simulink model "GraphicalFunction3_2018a"  (R2018a)
settings: Solver=FixedStepDiscrete  StartTime=0.0  StopTime=0.1  FixedStep=0.1  RelTol=1e-3  EnableMultiTasking=on
settings Model: Creator=bzhan  LastModifiedBy=bzhan
settings SolverCC: AutoInsertRateTranBlk=on
settings DataIOCC: LimitDataPoints=on  ReturnWorkspaceOutputs=on
settings OptimizationCC: LifeSpan=inf
settings DebuggingCC: AllowSymbolicDim=off  SFUnexpectedBacktrackingDiag=warning  SFNoUnconditionalDefaultTransitionDiag=warning  SFExecutionAtInitializationDiag=none
settings CodeAppCC: StateflowObjectComments=on
settings GRTTargetCC: TargetLangStandard=C89/C90 (ANSI)
settings ConfigComp: CovMetricSettings=dw  CovHtmlReporting=on  CovSaveCumulativeToWorkspaceVar=on  CovSaveSingleToWorkspaceVar=on  CovShowResultsExplorer=off  CovExternalEMLEnable=off  CovSFcnEnable=off

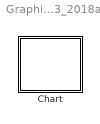
== system GraphicalFunction3_2018a ==
  Chart : Stateflow chart  TreatAsAtomicUnit=on

== stateflow chart GraphicalFunction3_2018a/Chart ==
  state index=find(N) [function]
    (junction 2) -> (junction 12) [order 3] : {index=i;}
    (default) -> (junction 2) : {i=1;}
    (junction 2) -> (junction 10) [order 2] : [i>N]
    (junction 10) -> (junction 12) : {index=-1;}
    (junction 2) -> (junction 5) [order 1] : [i<=N&&a(i)==0]
    (junction 6) -> (junction 2)
    (junction 5) -> (junction 6) : {i=i+1;}
  state [r,s]=square(i1,j1) [function]
    (default) -> (junction 30)
    (junction 30) -> (junction 33) : {r=i1*i1;}
    (junction 33) -> (junction 34) : {s=j1*j1;}
  state B
    en: f("en_B");
    [x,y]=square(x,y);
    g(x);g(y);
  state A
    en: f("en_A")
  (default) -> A
  A -> B : [find(4)==3]
  data: index function_output; N function_input; i1 function_input; j1 function_input; r function_output; s function_output; s function_input; n function_input; i local; x local double =2; y local double =3; a local =[0 0 1 2]
  function f(s):
    | function f(s)
    |   fprintf(s+"\n");
  function g(n):
    | function g(n)
    |   fprintf("%.0f\n", n);
